simulink model "CombEng"  (R2016a)
settings: Solver=FixedStepDiscrete  SolverMode=SingleTasking  StartTime=0.0  StopTime=inf  FixedStep=Ts  RelTol=1e-3
libraries: ArteChannelInterface_Lib_V1_2 x39, AVLArteLabLibrary x2, CommonLib x1, simulink x1
settings Model: Creator=luschana  LastModifiedBy=luschana
settings OptimizationCC: BlockReduction=off  OptimizeBlockIOStorage=off  BufferReuse=off  GlobalBufferReuse=off  ExpressionFolding=off  LocalBlockOutputs=off
settings RTWCC: SystemTargetFile=avl_artmi_intime6.tlc  MakeCommand=make_rtw_arte  TemplateMakefile=avl_artmivc.tmf  Description=Testbed.CONNECT Real Time Target (PO 2 R3)  CustomInclude=.  CustomSource=mexengine.cpp combustionengine.cpp cylinder.cpp definitions.cpp ecu.cpp environment.cpp gascomponent.cpp injector.cpp oil.cpp shomate.cpp valve.cpp  RTWCompilerOptimization=on
settings GRTTargetCC: CodeReplacementLibrary=GNU C99 extensions  GeneratePreprocessorConditionals=Use local settings  CombineOutputUpdateFcns=off  MatFileLogging=off  GRTInterface=on  UseToolchainInfoCompliant=off  RTWCAPISignals=on  RTWCAPIParams=on

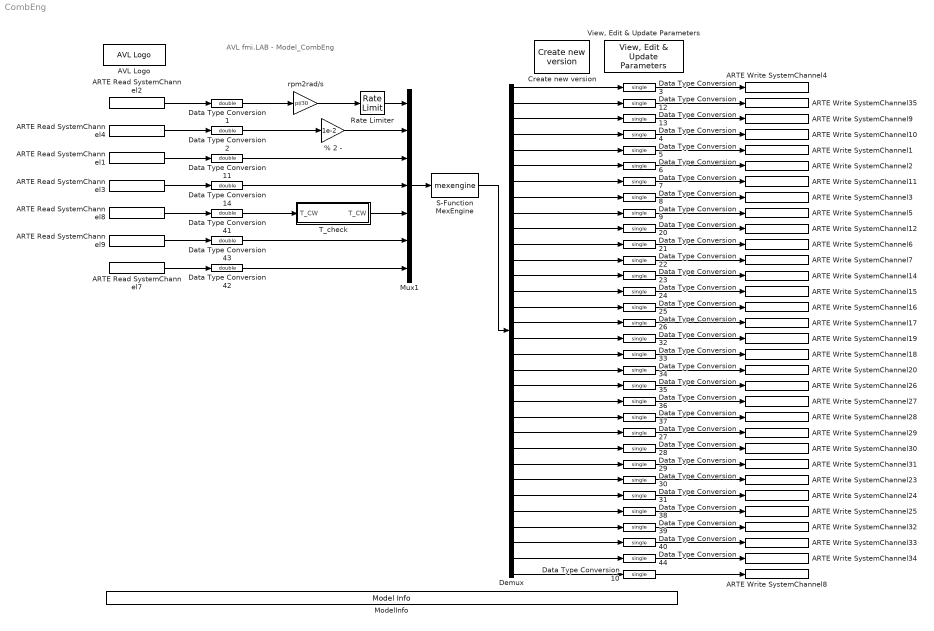
== system CombEng ==
  note: AVL fmi.LAB - Model_CombEng
  % 2 - : Gain  Gain=1e-2  ParamDataTypeStr=double  OutDataTypeStr=double
  ARTE Read SystemChannel1 : ArteChannelInterface_Lib_V1_2/ARTE Read SystemChannel  par1_name='SparkAngle'  type_idx=SystemVariable  par3_data_type=float  show_browser=off  hFig1=0  par6_status_chan=off  par5_mandatory=on  par7_ndf=off  par4_sample_time=Ts
  ARTE Read SystemChannel2 : ArteChannelInterface_Lib_V1_2/ARTE Read SystemChannel  par1_name='n_GBI'  type_idx=SystemVariable  par3_data_type=float  show_browser=off  hFig1=0  par6_status_chan=off  par5_mandatory=on  par7_ndf=off  par4_sample_time=Ts
  ARTE Read SystemChannel3 : ArteChannelInterface_Lib_V1_2/ARTE Read SystemChannel  par1_name='InjectionAngle'  type_idx=SystemVariable  par3_data_type=float  show_browser=off  hFig1=0  par6_status_chan=off  par5_mandatory=on  par7_ndf=off  par4_sample_time=Ts
  ARTE Read SystemChannel4 : ArteChannelInterface_Lib_V1_2/ARTE Read SystemChannel  par1_name='ThrPos_dem'  type_idx=SystemVariable  par3_data_type=float  show_browser=off  hFig1=0  par6_status_chan=off  par5_mandatory=on  par7_ndf=off  par4_sample_time=Ts
  ARTE Read SystemChannel7 : ArteChannelInterface_Lib_V1_2/ARTE Read SystemChannel  par1_name='amb_T'  type_idx=SystemVariable  par3_data_type=float  show_browser=off  hFig1=0  par6_status_chan=off  par5_mandatory=on  par7_ndf=off  par4_sample_time=Ts
  ARTE Read SystemChannel8 : ArteChannelInterface_Lib_V1_2/ARTE Read SystemChannel  par1_name='CW_T_out'  type_idx=SystemVariable  par3_data_type=float  show_browser=off  hFig1=0  par6_status_chan=off  par5_mandatory=on  par7_ndf=off  par4_sample_time=Ts
  ARTE Read SystemChannel9 : ArteChannelInterface_Lib_V1_2/ARTE Read SystemChannel  par1_name='amb_p'  type_idx=SystemVariable  par3_data_type=float  show_browser=off  hFig1=0  par6_status_chan=off  par5_mandatory=on  par7_ndf=off  par4_sample_time=Ts
  ARTE Write SystemChannel1 : ArteChannelInterface_Lib_V1_2/ARTE Write SystemChannel  par1_name='EngTemp'  type_idx=SystemVariable  par3_data_type=float  show_browser=off  hFig1=0  par4_status_chan=off
  ARTE Write SystemChannel10 : ArteChannelInterface_Lib_V1_2/ARTE Write SystemChannel  par1_name='freq_crankshaft'  type_idx=SystemVariable  par3_data_type=float  show_browser=off  hFig1=0  par4_status_chan=off
  ARTE Write SystemChannel11 : ArteChannelInterface_Lib_V1_2/ARTE Write SystemChannel  par1_name='intake_dot_n'  type_idx=SystemVariable  par3_data_type=float  show_browser=off  hFig1=0  par4_status_chan=off
  ARTE Write SystemChannel12 : ArteChannelInterface_Lib_V1_2/ARTE Write SystemChannel  par1_name='exhaust_dot_n'  type_idx=SystemVariable  par3_data_type=float  show_browser=off  hFig1=0  par4_status_chan=off
  ARTE Write SystemChannel14 : ArteChannelInterface_Lib_V1_2/ARTE Write SystemChannel  par1_name='exhaust_y_O2'  type_idx=SystemVariable  par3_data_type=float  show_browser=off  hFig1=0  par4_status_chan=off
  ARTE Write SystemChannel15 : ArteChannelInterface_Lib_V1_2/ARTE Write SystemChannel  par1_name='exhaust_y_H2O'  type_idx=SystemVariable  par3_data_type=float  show_browser=off  hFig1=0  par4_status_chan=off
  ARTE Write SystemChannel16 : ArteChannelInterface_Lib_V1_2/ARTE Write SystemChannel  par1_name='exhaust_y_CO2'  type_idx=SystemVariable  par3_data_type=float  show_browser=off  hFig1=0  par4_status_chan=off
  ARTE Write SystemChannel17 : ArteChannelInterface_Lib_V1_2/ARTE Write SystemChannel  par1_name='exhaust_y_CO'  type_idx=SystemVariable  par3_data_type=float  show_browser=off  hFig1=0  par4_status_chan=off
  ARTE Write SystemChannel18 : ArteChannelInterface_Lib_V1_2/ARTE Write SystemChannel  par1_name='exhaust_y_C'  type_idx=SystemVariable  par3_data_type=float  show_browser=off  hFig1=0  par4_status_chan=off
  ARTE Write SystemChannel19 : ArteChannelInterface_Lib_V1_2/ARTE Write SystemChannel  par1_name='exhaust_y_H2'  type_idx=SystemVariable  par3_data_type=float  show_browser=off  hFig1=0  par4_status_chan=off
  ARTE Write SystemChannel2 : ArteChannelInterface_Lib_V1_2/ARTE Write SystemChannel  par1_name='dot_n_Fuel'  type_idx=SystemVariable  par3_data_type=float  show_browser=off  hFig1=0  par4_status_chan=off
  ARTE Write SystemChannel20 : ArteChannelInterface_Lib_V1_2/ARTE Write SystemChannel  par1_name='exhaust_y_Fuel'  type_idx=SystemVariable  par3_data_type=float  show_browser=off  hFig1=0  par4_status_chan=off
  ARTE Write SystemChannel23 : ArteChannelInterface_Lib_V1_2/ARTE Write SystemChannel  par1_name='Cyl1_T'  type_idx=SystemVariable  par3_data_type=float  show_browser=off  hFig1=0  par4_status_chan=off
  ARTE Write SystemChannel24 : ArteChannelInterface_Lib_V1_2/ARTE Write SystemChannel  par1_name='Cyl2_T'  type_idx=SystemVariable  par3_data_type=float  show_browser=off  hFig1=0  par4_status_chan=off
  ARTE Write SystemChannel25 : ArteChannelInterface_Lib_V1_2/ARTE Write SystemChannel  par1_name='Cyl3_T'  type_idx=SystemVariable  par3_data_type=float  show_browser=off  hFig1=0  par4_status_chan=off
  ARTE Write SystemChannel26 : ArteChannelInterface_Lib_V1_2/ARTE Write SystemChannel  par1_name='Cyl1_p'  type_idx=SystemVariable  par3_data_type=float  show_browser=off  hFig1=0  par4_status_chan=off
  ARTE Write SystemChannel27 : ArteChannelInterface_Lib_V1_2/ARTE Write SystemChannel  par1_name='Cyl2_p'  type_idx=SystemVariable  par3_data_type=float  show_browser=off  hFig1=0  par4_status_chan=off
  ARTE Write SystemChannel28 : ArteChannelInterface_Lib_V1_2/ARTE Write SystemChannel  par1_name='Cyl3_p'  type_idx=SystemVariable  par3_data_type=float  show_browser=off  hFig1=0  par4_status_chan=off
  ARTE Write SystemChannel29 : ArteChannelInterface_Lib_V1_2/ARTE Write SystemChannel  par1_name='Cyl4_p'  type_idx=SystemVariable  par3_data_type=float  show_browser=off  hFig1=0  par4_status_chan=off
  ARTE Write SystemChannel3 : ArteChannelInterface_Lib_V1_2/ARTE Write SystemChannel  par1_name='intake_p'  type_idx=SystemVariable  par3_data_type=float  show_browser=off  hFig1=0  par4_status_chan=off
  ARTE Write SystemChannel30 : ArteChannelInterface_Lib_V1_2/ARTE Write SystemChannel  par1_name='Cyl5_p'  type_idx=SystemVariable  par3_data_type=float  show_browser=off  hFig1=0  par4_status_chan=off
  ARTE Write SystemChannel31 : ArteChannelInterface_Lib_V1_2/ARTE Write SystemChannel  par1_name='Cyl6_p'  type_idx=SystemVariable  par3_data_type=float  show_browser=off  hFig1=0  par4_status_chan=off
  ARTE Write SystemChannel32 : ArteChannelInterface_Lib_V1_2/ARTE Write SystemChannel  par1_name='Cyl4_T'  type_idx=SystemVariable  par3_data_type=float  show_browser=off  hFig1=0  par4_status_chan=off
  ARTE Write SystemChannel33 : ArteChannelInterface_Lib_V1_2/ARTE Write SystemChannel  par1_name='Cyl5_T'  type_idx=SystemVariable  par3_data_type=float  show_browser=off  hFig1=0  par4_status_chan=off
  ARTE Write SystemChannel34 : ArteChannelInterface_Lib_V1_2/ARTE Write SystemChannel  par1_name='Cyl6_T'  type_idx=SystemVariable  par3_data_type=float  show_browser=off  hFig1=0  par4_status_chan=off
  ARTE Write SystemChannel35 : ArteChannelInterface_Lib_V1_2/ARTE Write SystemChannel  par1_name='CW_dotQ_Cooling'  type_idx=SystemVariable  par3_data_type=float  show_browser=off  hFig1=0  par4_status_chan=off
  ARTE Write SystemChannel4 : ArteChannelInterface_Lib_V1_2/ARTE Write SystemChannel  par1_name='T_crankshaft'  type_idx=SystemVariable  par3_data_type=float  show_browser=off  hFig1=0  par4_status_chan=off
  ARTE Write SystemChannel5 : ArteChannelInterface_Lib_V1_2/ARTE Write SystemChannel  par1_name='intake_T'  type_idx=SystemVariable  par3_data_type=float  show_browser=off  hFig1=0  par4_status_chan=off
  ARTE Write SystemChannel6 : ArteChannelInterface_Lib_V1_2/ARTE Write SystemChannel  par1_name='exhaust_p'  type_idx=SystemVariable  par3_data_type=float  show_browser=off  hFig1=0  par4_status_chan=off
  ARTE Write SystemChannel7 : ArteChannelInterface_Lib_V1_2/ARTE Write SystemChannel  par1_name='exhaust_T'  type_idx=SystemVariable  par3_data_type=float  show_browser=off  hFig1=0  par4_status_chan=off
  ARTE Write SystemChannel8 : ArteChannelInterface_Lib_V1_2/ARTE Write SystemChannel  par1_name='Env_out_T'  type_idx=SystemVariable  par3_data_type=float  show_browser=off  hFig1=0  par4_status_chan=off
  ARTE Write SystemChannel9 : ArteChannelInterface_Lib_V1_2/ARTE Write SystemChannel  par1_name='phi_crankshaft'  type_idx=SystemVariable  par3_data_type=float  show_browser=off  hFig1=0  par4_status_chan=off
  AVL Logo : CommonLib/CommonLib/AVL Logo  SystemSampleTime=-1
  Create new version : AVLArteLabLibrary/Create new version
  Data Type Conversion{1..2,11,14,41..43} (7 alike) : DataTypeConversion  OutDataTypeStr=double
  Data Type Conversion{3..10,12..13,20..40,44} (32 alike) : DataTypeConversion  OutDataTypeStr=single
  Demux : Demux  Outputs=32
  ModelInfo : simulink/Model-Wide Utilities/Model Info  Frame=on  DisplayStringWithTags=Modified by: %<ModifiedBy>; Model Version: %<ModelVersion>; Last Modified: %<LastModificationDate>  HorizontalTextAlignment=Center  LeftAlignmentValue=0.5  SourceBlockDiagram=CombEng  TagMaxNumber=20
  Mux1 : Mux  Inputs=7
  Rate Limiter : RateLimiter  RisingSlewLimit=1000  FallingSlewLimit=-1000  SampleTimeMode=inherited
  S-Function MexEngine : S-Function  FunctionName=mexengine  SFunctionModules='combustionengine cylinder definitions ecu environment gascomponent shomate valve'  SFunctionDeploymentMode=off  EnableBusSupport=off
  T_check : MATLAB Function  TreatAsAtomicUnit=on
  "View, Edit & Update Parameters" : AVLArteLabLibrary/View, Edit & Update Parameters
  "rpm2rad/s " : Gain  Gain=pi/30  ParamDataTypeStr=double  OutDataTypeStr=double
  wires:
  Data Type Conversion1/1 -> "rpm2rad/s "/1
  "rpm2rad/s "/1 -> Rate Limiter/1
  Data Type Conversion2/1 -> % 2 -/1
  % 2 -/1 -> Mux1/2
  Rate Limiter/1 -> Mux1/1
  Mux1/1 -> S-Function MexEngine/1
  S-Function MexEngine/1 -> Demux/1
  ARTE Read SystemChannel2/1 -> Data Type Conversion1/1
  ARTE Read SystemChannel4/1 -> Data Type Conversion2/1
  Data Type Conversion3/1 -> ARTE Write SystemChannel4/1
  Data Type Conversion4/1 -> ARTE Write SystemChannel10/1
  Data Type Conversion5/1 -> ARTE Write SystemChannel1/1
  Data Type Conversion6/1 -> ARTE Write SystemChannel2/1
  Data Type Conversion7/1 -> ARTE Write SystemChannel11/1
  Data Type Conversion11/1 -> Mux1/3
  ARTE Read SystemChannel1/1 -> Data Type Conversion11/1
  Data Type Conversion12/1 -> ARTE Write SystemChannel35/1
  Demux/1 -> Data Type Conversion3/1
  Demux/2 -> Data Type Conversion12/1
  Data Type Conversion13/1 -> ARTE Write SystemChannel9/1
  Demux/3 -> Data Type Conversion13/1
  Demux/4 -> Data Type Conversion4/1
  Demux/5 -> Data Type Conversion5/1
  Demux/6 -> Data Type Conversion6/1
  Demux/7 -> Data Type Conversion7/1
  Data Type Conversion9/1 -> ARTE Write SystemChannel5/1
  Demux/8 -> Data Type Conversion8/1
  Demux/9 -> Data Type Conversion9/1
  Data Type Conversion8/1 -> ARTE Write SystemChannel3/1
  Data Type Conversion20/1 -> ARTE Write SystemChannel12/1
  Data Type Conversion21/1 -> ARTE Write SystemChannel6/1
  Data Type Conversion22/1 -> ARTE Write SystemChannel7/1
  Data Type Conversion23/1 -> ARTE Write SystemChannel14/1
  Data Type Conversion25/1 -> ARTE Write SystemChannel16/1
  Data Type Conversion24/1 -> ARTE Write SystemChannel15/1
  Data Type Conversion26/1 -> ARTE Write SystemChannel17/1
  Data Type Conversion34/1 -> ARTE Write SystemChannel20/1
  Data Type Conversion35/1 -> ARTE Write SystemChannel26/1
  Data Type Conversion37/1 -> ARTE Write SystemChannel28/1
  Data Type Conversion36/1 -> ARTE Write SystemChannel27/1
  Demux/10 -> Data Type Conversion20/1
  Demux/11 -> Data Type Conversion21/1
  Demux/12 -> Data Type Conversion22/1
  Demux/13 -> Data Type Conversion23/1
  Demux/14 -> Data Type Conversion24/1
  Demux/15 -> Data Type Conversion25/1
  Demux/16 -> Data Type Conversion26/1
  Data Type Conversion27/1 -> ARTE Write SystemChannel29/1
  Data Type Conversion28/1 -> ARTE Write SystemChannel30/1
  Demux/22 -> Data Type Conversion37/1
  Demux/17 -> Data Type Conversion32/1
  Demux/18 -> Data Type Conversion33/1
  Demux/19 -> Data Type Conversion34/1
  Demux/20 -> Data Type Conversion35/1
  Demux/21 -> Data Type Conversion36/1
  Data Type Conversion29/1 -> ARTE Write SystemChannel31/1
  Data Type Conversion30/1 -> ARTE Write SystemChannel23/1
  Data Type Conversion31/1 -> ARTE Write SystemChannel24/1
  Data Type Conversion38/1 -> ARTE Write SystemChannel25/1
  Data Type Conversion40/1 -> ARTE Write SystemChannel33/1
  Data Type Conversion39/1 -> ARTE Write SystemChannel32/1
  Demux/26 -> Data Type Conversion30/1
  Demux/25 -> Data Type Conversion29/1
  Demux/28 -> Data Type Conversion38/1
  Demux/29 -> Data Type Conversion39/1
  Demux/27 -> Data Type Conversion31/1
  Demux/30 -> Data Type Conversion40/1
  ARTE Read SystemChannel8/1 -> Data Type Conversion41/1
  ARTE Read SystemChannel9/1 -> Data Type Conversion43/1
  ARTE Read SystemChannel7/1 -> Data Type Conversion42/1
  Data Type Conversion44/1 -> ARTE Write SystemChannel34/1
  Demux/31 -> Data Type Conversion44/1
  Demux/23 -> Data Type Conversion27/1
  Demux/24 -> Data Type Conversion28/1
  Data Type Conversion41/1 -> T_check/1("T_CW ")
  Data Type Conversion10/1 -> ARTE Write SystemChannel8/1
  Demux/32 -> Data Type Conversion10/1
  ARTE Read SystemChannel3/1 -> Data Type Conversion14/1
  Data Type Conversion14/1 -> Mux1/4
  T_check/1(T_CW) -> Mux1/5
  Data Type Conversion43/1 -> Mux1/6
  Data Type Conversion42/1 -> Mux1/7
  Data Type Conversion33/1 -> ARTE Write SystemChannel18/1
  Data Type Conversion32/1 -> ARTE Write SystemChannel19/1

== matlab function CombEng/T_check ==
  settings: updateMethod=DISCRETE  sampleTime=Ts
  data: T_CW output; T_CW input double
function T_CW  = calc(T_CW)
if(T_CW < 250.0)
    T_CW = 330;
end
if(T_CW > 500.0)
    T_CW = 500;
end
